simulink model "lab1"  (R2020a)
settings: Solver=FixedStepDiscrete  StartTime=0.0  StopTime=10.0  RelTol=1e-3
libraries: dspsigops x2, dsparch4 x1, dspspect3 x1
settings Model: Creator=mawil  LastModifiedBy=mawil

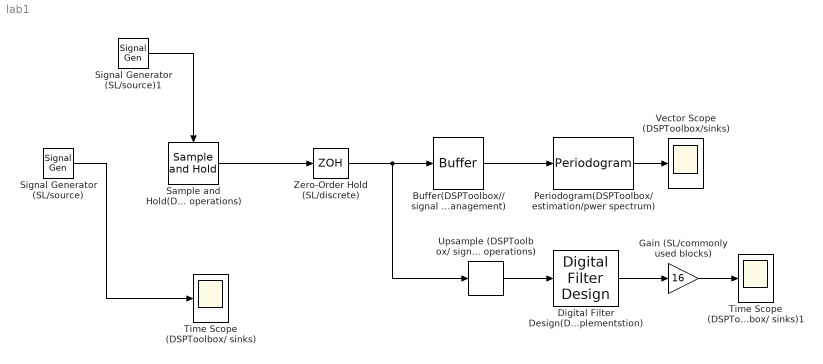
== system lab1 ==
  Buffer(DSPToolbox// signal management) : Buffer  N=256
  Digital Filter Design(DSPToolbox/Fitering/ Filter Implementstion) : dsparch4/Digital Filter Design  mwdsp_browser_bugfix_var=off
  Gain (SL/commonly used blocks) : Gain  Gain=16
  Periodogram(DSPToolbox/ estimation/pwer spectrum) : dspspect3/Periodogram  measurement=Power spectral density  wintype=Hamming  Rs=50  beta=5  winsamp=Symmetric  FFTImplementation=Auto  inheritFFT=off  fftsize=256  navg=4  inheritTs=on  Ts=1
      settings: SourceProductBaseCode=DS
  Sample and Hold(DSPToolbox /signal operations) : dspsigops/Sample and Hold  trig=Rising edge  initCond=0  latchinput=off
  Signal Generator (SL/source) : SignalGenerator  Frequency=100
  Signal Generator (SL/source)1 : SignalGenerator  WaveForm=square  Frequency=1000
  Time Scope (DSPToolbox/ sinks) : Scope
  Time Scope (DSPToolbox/ sinks)1 : Scope
  Upsample (DSPToolbox/ signal operations) : dspsigops/Upsample  N=16  phase=0  InputProcessing=Columns as channels (frame based)  RateOptions=Enforce single-rate processing  ic=0  mode=Unused parameter value
  Vector Scope (DSPToolbox/sinks) : Scope
  Zero-Order Hold (SL/discrete) : ZeroOrderHold
  wires:
  Signal Generator (SL/source)/1 -> Time Scope (DSPToolbox/ sinks)/1
  Signal Generator (SL/source)1/1 -> Sample and Hold(DSPToolbox /signal operations)/Trigger
  Sample and Hold(DSPToolbox /signal operations)/1 -> Zero-Order Hold (SL/discrete)/1
  Zero-Order Hold (SL/discrete)/1 -> Buffer(DSPToolbox// signal management)/1, Upsample (DSPToolbox/ signal operations)/1
  Periodogram(DSPToolbox/ estimation/pwer spectrum)/1 -> Vector Scope (DSPToolbox/sinks)/1
  Buffer(DSPToolbox// signal management)/1 -> Periodogram(DSPToolbox/ estimation/pwer spectrum)/1
  Upsample (DSPToolbox/ signal operations)/1 -> Digital Filter Design(DSPToolbox/Fitering/ Filter Implementstion)/1
  Digital Filter Design(DSPToolbox/Fitering/ Filter Implementstion)/1 -> Gain (SL/commonly used blocks)/1
  Gain (SL/commonly used blocks)/1 -> Time Scope (DSPToolbox/ sinks)1/1
